simulink model "sequence_dwa_obstacle_avoidance"  (R2023b)
settings: Solver=VariableStepAuto  StartTime=0.0  StopTime=250  RelTol=1e-3
values from neighbouring files (symbols this model uses):
  initTheta = 0    [dynamic_window_init.m]    (also in sequence_dynamic_window_init.m; sequence_visualize.m = out.pose(1,3); visualize.m = out.pose(1,3))
  initX = 6    [dynamic_window_init.m]    (also in sequence_dynamic_window_init.m = 36; sequence_visualize.m = out.pose(1,1); visualize.m = out.pose(1,1))
  initY = 21    [dynamic_window_init.m]    (also in sequence_dynamic_window_init.m = 34; sequence_visualize.m = out.pose(1,2); visualize.m = out.pose(1,2))
  k1 = 0.80    (= 0.8)    [dynamic_window_init.m]    (also in sequence_dynamic_window_init.m = 0.9)
  k2 = 0.006    [dynamic_window_init.m]    (also in sequence_dynamic_window_init.m)
  k3 = 0.02    [dynamic_window_init.m]    (also in sequence_dynamic_window_init.m = 0.1)
  mapMatrix = map2    [dynamic_window_init.m]    (also in sequence_dynamic_window_init.m = map3)
  mapScale = 1    [dynamic_window_init.m]    (also in sequence_dynamic_window_init.m)
  maxLinSpeed = 1.5    [dynamic_window_init.m]    (also in sequence_dynamic_window_init.m)
  maxRange = 12    [dynamic_window_init.m]    (also in sequence_dynamic_window_init.m)
  sampleTime = 0.05    [dynamic_window_init.m]    (also in sequence_dynamic_window_init.m)
  targets = [58,49 ... (first row only)    [sequence_dynamic_window_init.m]
  v0 = 0    [dynamic_window_init.m]    (also in sequence_dynamic_window_init.m)
  w0 = 0    [dynamic_window_init.m]    (also in sequence_dynamic_window_init.m)
libraries: robotmobilelib x1
settings Model: SnapshotBufferSize=100  Creator=lucia  LastModifiedBy=lucia

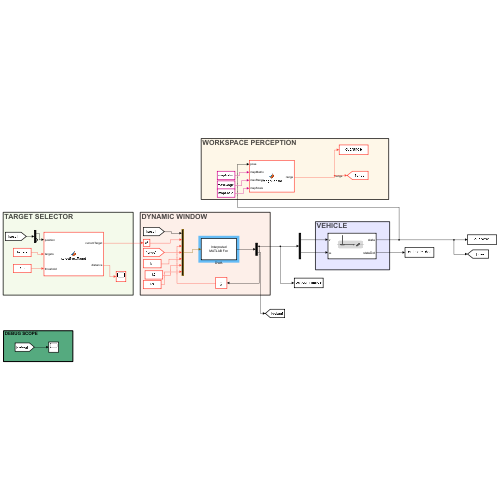
[thumbnail: Simulink's stored preview of the top-level diagram]
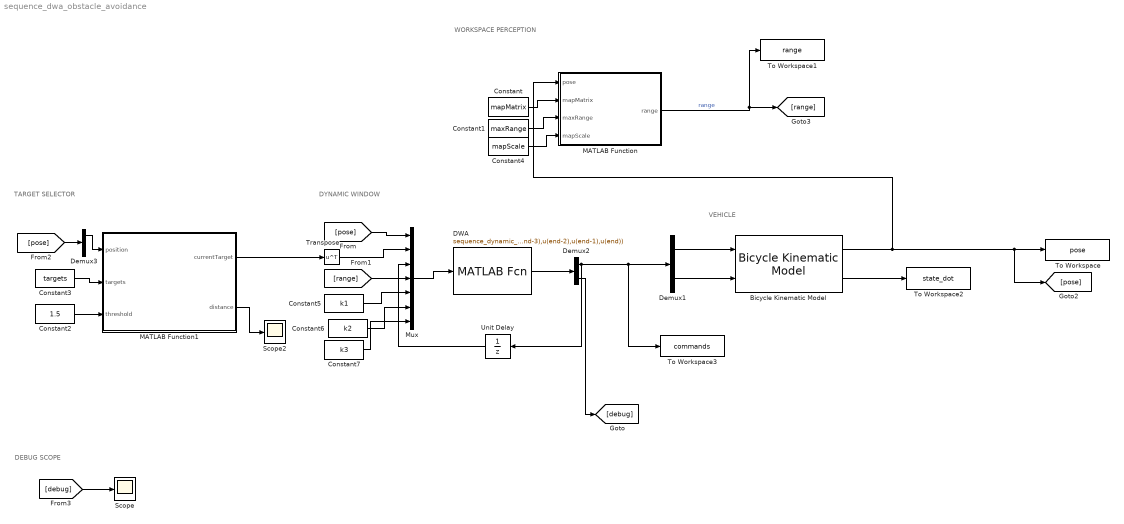
== system sequence_dwa_obstacle_avoidance ==
  note: DEBUG SCOPE
  note: DYNAMIC WINDOW
  note: VEHICLE
  note: WORKSPACE PERCEPTION
  note: TARGET SELECTOR
  Bicycle Kinematic Model : robotmobilelib/Bicycle Kinematic Model  VehicleInputs=Vehicle Speed & Heading Angular Velocity  WheelBase=wheelBase  VehicleSpeedRange=[0 maxLinSpeed]  MaxSteeringAngle=maxAngle  InitialState=[initX, initY, initTheta]  SimulateUsing=Interpreted execution
  Constant : Constant  Value=mapMatrix
  Constant1 : Constant  Value=maxRange
  Constant2 : Constant  Value=1.5  SampleTime=sampleTime
  Constant3 : Constant  Value=targets  SampleTime=sampleTime
  Constant4 : Constant  Value=mapScale
  Constant5 : Constant  Value=k1  SampleTime=sampleTime
  Constant6 : Constant  Value=k2  SampleTime=sampleTime
  Constant7 : Constant  Value=k3  SampleTime=sampleTime
  DWA : MATLABFcn  MATLABFcn=sequence_dynamic_window(u(1:3),u(4:5),u(6:7),u(8:end-3),u(end-2),u(end-1),u(end))  OutputDimensions=5
  Demux1 : Demux  Outputs=2
  Demux2 : Demux  Outputs=[2 3]
  Demux3 : Demux  Outputs=[2 1]
  MATLAB Function : MATLAB Function  TreatAsAtomicUnit=on
  MATLAB Function1 : MATLAB Function  TreatAsAtomicUnit=on
  Mux : Mux  Inputs=7
  Scope : Scope
  Scope2 : Scope
  To Workspace : ToWorkspace  VariableName=pose  SampleTime=-1
      settings: Save2DSignal=2-D array (concatenate along first dimension)
  To Workspace1 : ToWorkspace  VariableName=range  SampleTime=-1
  To Workspace2 : ToWorkspace  VariableName=state_dot  SampleTime=-1
      settings: Save2DSignal=2-D array (concatenate along first dimension)
  To Workspace3 : ToWorkspace  VariableName=commands  SampleTime=-1
      settings: Save2DSignal=2-D array (concatenate along first dimension)
  Transpose : Math  Operator=transpose
  Unit Delay : UnitDelay  InitialCondition=[v0; w0]  SampleTime=sampleTime  HasFrameUpgradeWarning=on
  wires:
  Bicycle Kinematic Model/1 -> [pose], To Workspace/1, MATLAB Function/1(pose)
  Constant1/1 -> MATLAB Function/3(maxRange)
  Constant/1 -> MATLAB Function/2(mapMatrix)
  DWA/1 -> Demux2/1
  [pose] -> Mux/1
  [range] -> Mux/4
  Unit Delay/1 -> Mux/3
  MATLAB Function1/1(currentTarget) -> Transpose/1
  Bicycle Kinematic Model/2 -> To Workspace2/1
  Demux2/1 -> Unit Delay/1, Demux1/1, To Workspace3/1
  Demux1/1 -> Bicycle Kinematic Model/1
  Mux/1 -> DWA/1
  MATLAB Function/1(range) -> To Workspace1/1, [range]  "range"
  Demux1/2 -> Bicycle Kinematic Model/2
  Constant3/1 -> MATLAB Function1/2(targets)
  Constant2/1 -> MATLAB Function1/3(threshold)
  Transpose/1 -> Mux/2
  [pose] -> Demux3/1
  Demux3/1 -> MATLAB Function1/1(position)
  MATLAB Function1/2(distance) -> Scope2/1
  Constant4/1 -> MATLAB Function/4(mapScale)
  Demux2/2 -> [debug]
  [debug] -> Scope/1
  Constant5/1 -> Mux/5
  Constant6/1 -> Mux/6
  Constant7/1 -> Mux/7

== matlab function sequence_dwa_obstacle_avoidance/MATLAB Function ==
  settings: updateMethod=DISCRETE
  data: range output size=[129,1]; pose input size=[3, 1]; mapMatrix input size=[size(mapMatrix, 1), size(mapMatrix, 2)]; maxRange input; mapScale input
function range = RangeSensor(pose, mapMatrix, maxRange, mapScale)
% This function may be removed in the future.
% Copyright The MathWorks Inc, 2023
persistent r
 if isempty(r)
    r = rangeSensor('HorizontalAngle', [-pi/2,pi/2], 'HorizontalAngleResolution', pi/128, 'Range', [0 maxRange]);
end
map = binaryOccupancyMap(mapMatrix, 1);
p = pose';

% The range sensor accepts a pose on the map which is within the map's
% limits. Thus, filter out positions outside the map, and override them
% with readings that are zero.
xcord=p(:,1);
ycord=p(:,2);
xmin=map.XWorldLimits(1);
ymin=map.YWorldLimits(1);
xmax=map.XWorldLimits(2);
ymax=map.YWorldLimits(2);
isxvalid=xcord>=xmin&xcord<=xmax;
isyvalid=ycord>=ymin&ycord<=ymax;
isInside=isxvalid&isyvalid;
range = zeros(r.NumReadings,size(p,1));
range(:,isInside) = r(p(isInside,:), map);
%angles = -3*pi/8:pi/8:3*pi/8
end

== matlab function sequence_dwa_obstacle_avoidance/MATLAB Function1 ==
  settings: updateMethod=DISCRETE
  data: position input; currentTarget output; targets input; threshold input; distance output
function [currentTarget, distance] = selectNextTarget(position, targets, threshold)
    % position: posizione corrente del robot [x, y]
    % targets: matrice con i target [x1, y1; x2, y2; ...]
    % targetIndex: indice del target corrente
    % threshold: distanza per considerare il target raggiunto

    persistent targetIndex
    if isempty(targetIndex)
        targetIndex=1;
    end
    % Ottieni il target corrente
    currentTarget = targets(targetIndex, :);
    
    % Calcola la distanza dal target corrente
    distance = sqrt((position(1)-currentTarget(1))^2+(position(2)-currentTarget(2))^2);
    
    % Controlla se il target è stato raggiunto
    if distance < threshold
        % Passa al target successivo, se esiste
        if targetIndex < size(targets, 1)
            targetIndex = targetIndex + 1;
        else
            % Resta sull'ultimo target se non ci sono altri
            targetIndex = size(targets, 1);
        end
    end
    
    % Aggiorna il target corrente
    currentTarget = targets(targetIndex, :);
end
